simulink model "Tricycle_EKF_Pose_estimation"  (R2020b)
settings: Solver=FixedStepDiscrete  StartTime=0.0  StopTime=50  FixedStep=0.02  RelTol=1e-3  EnableMultiTasking=on
InitFcn:
  | ProcNoiseD=0.01^2; % is a variance
  | ProcNoiseTheta=0.001^2; % is a variance
  | Ts=0.1
undefined symbols (not defined in the file or in its folder): V
settings Model: Creator=antonio  LastModifiedBy=antonio
settings DataIOCC: LimitDataPoints=on  SaveFormat=Array  ReturnWorkspaceOutputs=off
settings OptimizationCC: LifeSpan=inf
settings DebuggingCC: UnderspecifiedInitializationDetection=Classic  MergeDetectMultiDrivingBlocksExec=none  SolverPrmCheckMsg=warning  StateNameClashWarn=warning  SFUnexpectedBacktrackingDiag=warning  SFNoUnconditionalDefaultTransitionDiag=warning  SFExecutionAtInitializationDiag=none  ArithmeticOperatorsInVariantConditions=warning
settings HardwareCC: ProdBitPerPointer=32  ProdBitPerSizeT=32  ProdBitPerPtrDiffT=32  ProdLargestAtomicFloat=None  ProdIntDivRoundTo=Undefined  ProdEndianess=Unspecified  ProdWordSize=32  ProdHWDeviceType=32-bit Generic
settings ModelReferenceCC: PropagateSignalLabelsOutOfModel=off
settings SFSimCC: SimUseLocalCustomCode=off  CustomCodeUndefinedFunction=UseInterfaceOnly
settings RTWCC: RTWUseLocalCustomCode=off
settings CodeAppCC: StateflowObjectComments=on
settings GRTTargetCC: TargetLangStandard=C89/C90 (ANSI)
settings ConfigComp: CovMetricSettings=dw  CovSaveCumulativeToWorkspaceVar=on  CovSaveSingleToWorkspaceVar=on  CovExternalEMLEnable=off

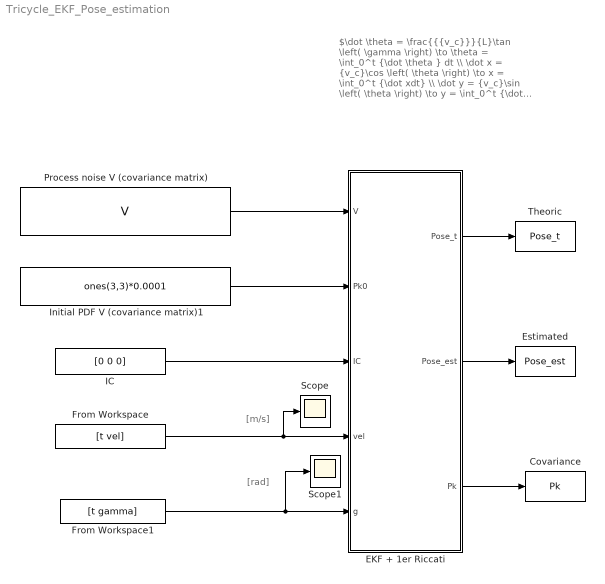
== system Tricycle_EKF_Pose_estimation ==
  note: $\dot \theta = \frac{{{v_c}}}{L}\tan \left( \gamma \right) \to \theta = \int_0^t {\dot \theta } dt \\ \dot x = {v_c}\cos \left( \theta \right) \to x = \int_0^t {\dot xdt} \\ \dot y = {v_c}\sin \left( \theta \right) \to y = \int_0^t {\dot ydt} \\ \end{gathered} \]$
  note: [rad]
  note: [m/s]
  Covariance : ToWorkspace  VariableName=Pk  SaveFormat=Structure With Time  SampleTime=-1
  EKF + 1er Riccati : MATLAB Function  TreatAsAtomicUnit=on
  Estimated : ToWorkspace  VariableName=Pose_est  SaveFormat=Timeseries  SampleTime=-1
  From Workspace : FromWorkspace  VariableName=[t vel]  SampleTime=Ts
  From Workspace1 : FromWorkspace  VariableName=[t gamma]  SampleTime=Ts
  IC : Constant  Value=[0 0 0]
  Initial PDF V (covariance matrix)1 : Constant  Value=ones(3,3)*0.0001  VectorParams1D=off
  Process noise V (covariance matrix) : Constant  Value=V  VectorParams1D=off
  Scope : Scope
  Scope1 : Scope
  Theoric : ToWorkspace  VariableName=Pose_t  SaveFormat=Timeseries  SampleTime=-1
  wires:
  IC/1 -> EKF + 1er Riccati/3(IC)
  EKF + 1er Riccati/1(Pose_t) -> Theoric/1
  EKF + 1er Riccati/2(Pose_est) -> Estimated/1
  From Workspace1/1 -> Scope1/1, EKF + 1er Riccati/5(g)
  From Workspace/1 -> Scope/1, EKF + 1er Riccati/4(vel)
  Process noise V (covariance matrix)/1 -> EKF + 1er Riccati/1(V)
  Initial PDF V (covariance matrix)1/1 -> EKF + 1er Riccati/2(Pk0)
  EKF + 1er Riccati/3(Pk) -> Covariance/1

== matlab function Tricycle_EKF_Pose_estimation/EKF + 1er Riccati ==
  data: V input; Pk0 input; Pose_t output; Pose_est output; IC input; vel input; g input; Pk output
function [Pose_t,Pose_est,Pk] = fcn(V,Pk0,IC,vel,g) % IC->Initial Condition [xo,yo,th0]
                                   % R and L are the displacements of
                                   % wheels [m]
persistent x_w y_w suma_theta...%  internal variable to be mantain its values
           Pose_est1 Pk1

ts=0.1; % sample time
L = 1;

%%%%%%%%%%%%%%%%%%%%%%%%%%%%%%%%%%%%%%%%%%%%%%%%%%%%%%%%%%%%%%%%%%%%%%%%%%
% %%%%%%%%%%%%%%   Read Initial condition   %%%%%%%%%%%%%%%%%%%%%%%%%%%%%%
x_ini=IC(1);
y_ini=IC(2);
theta_ini=IC(3);
P_ini=Pk0;

%%%%%%%%%%%%%%%%%%%%%%%%%%%%%%%%%%%%%%%%%%%%%%%%%%%%%%%%%%%%%%%%%%%%%%%%%%
%%%%%%%%%%%%%%%   variable initialitation  %%%%%%%%%%%%%%%%%%%%%%%%%%%%%%
if isempty (x_w)
    x_w=x_ini;
    y_w=y_ini;
    suma_theta=theta_ini; 
    Pose_est1 = [x_w;y_w;suma_theta];
    %Pose_t=[x_w;y_w;suma_theta]
    Pk1 = P_ini;
end

%%%%%%%%%%%%%%%%%%%%%%%%%%%%%%%%%%%%%%%%%%%%%%%%%%%%%%%%%%%%%%%%%%%%%%%%%%
%%%%%%%%%%%%%%%%%  Compute the odometry    %%%%%%%%%%%%%%%%%%%%%%%%%%%%%%%
delta_th = ts*vel*tan(g)/L;
delta_d = vel*ts;
%%%%%%%%%%%%%%%%%%%%%%%%%%%%%%%%%%%%%%%%%%%%%%%%%%%%%%%%%%%%%%%%%%%%%%%%%%
%%%%%%%%%%%%%%%%%  integration of the robot pose %%%%%%%%%%%%%%%%%%%%%%%%%%
suma_theta=mod((suma_theta+delta_th),2*pi);
x_w = x_w + (delta_d *cos(suma_theta));
y_w = y_w + (delta_d *sin(suma_theta));
Pose_t=[x_w;y_w;suma_theta];

%%%%%%%%%%%%%%%%%%%%%%%%%%%%%%%%%%%%%%%%%%%%%%%%%%%%%%%%%%%%%%%%%%%%%%%%%%
%%%%%%%%%%%%%%%%%  Build the Jacocian %%%%%%%%%%%%%%%%%%%%%%%%%%%%%%%%%%%%3

F_x = [[1 0 -(delta_d*sin(suma_theta+delta_th))];....
      [0 1 -(delta_d*cos(suma_theta+delta_th))];....
      [0 0 1]];

F_v = [[cos(suma_theta+delta_th) -delta_d*sin(suma_theta+delta_th)];....
      [sin(suma_theta+delta_th) delta_d*cos(suma_theta+delta_th)];[0 1]];

%%%%%%%%%%%%%%%%%%%%%%%%%%%%%%%%%%%%%%%%%%%%%%%%%%%%%%%%%%%%%%%%%%%%%%%%%%
%%%%%%%%%%%%%%%%% Compute the EKF Trucated Taylor %%%%%%%%%%%%%%%%%%%%%%%%

Pose_est1 = Pose_est1 + F_x*(Pose_t - Pose_est1) + F_v*diag(V);

Pk1 = F_x*Pk1*F_x' + F_v*V*F_v';

%%%%%%%%%%%%%%%%%%%%%%%%%%%%%%%%%%%%%%%%%%%%%%%%%%%%%%%%%%%%%%%%%%%%%%%%%%
%%%%%%%%%%%%%%%%%  output variable %%%%%%%%%%%%%%%%%%%%%%%%%%%%%%%%%%%%%%%

Pose_t=[x_w;y_w;suma_theta];
Pose_est= Pose_est1;
Pk=Pk1;

end
